simulink model "simpleSwitchWithSubsystemIn"  (R2025a)
settings: Solver=ode4  StartTime=0.0  StopTime=10.0  FixedStep=0.1  RelTol=1e-3
model workspace (MAT data in the model file):
  Bias1 = -2
  Bias2 = -2
  Bias3 = -2
  Bias4 = -2
libraries: simulink x2
settings Model: Creator=The MathWorks, Inc.  LastModifiedBy=The MathWorks, Inc.
settings SolverCC: AlgebraicLoopSolver=TrustRegion
settings DataIOCC: SaveTime=off
settings DebuggingCC: UnconnectedInputMsg=warning  UnconnectedOutputMsg=warning  UnconnectedLineMsg=warning
settings ModelReferenceCC: EnableRefExpFcnMdlSchedulingChecks=on
settings RTWCC: GPUComputeCapability=3.5  DLArmComputeVersion=19.05

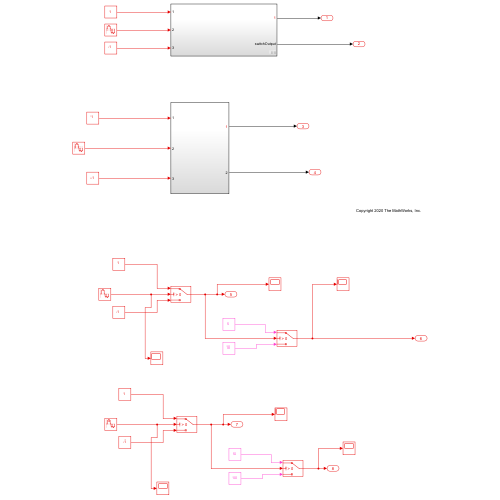
[thumbnail: Simulink's stored preview of the top-level diagram]
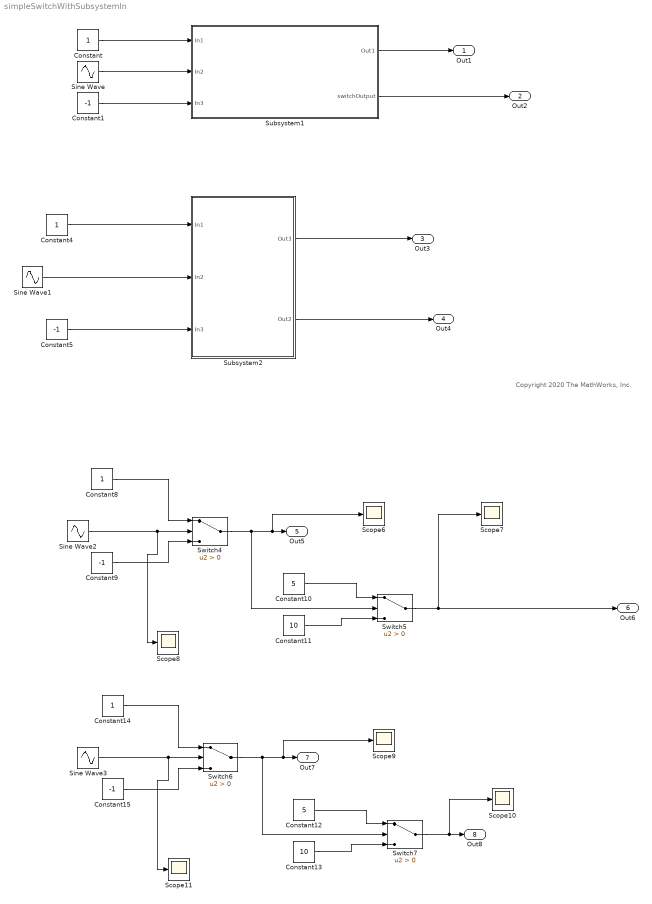
== system simpleSwitchWithSubsystemIn ==
  note: Copyright 2020 The MathWorks, Inc.
  Constant{,4,8,14} (4 alike) : Constant  SampleTime=0.1
  Constant{1,5,9,15} (4 alike) : Constant  Value=-1  SampleTime=0.1
  Constant10 : Constant  Value=5
  Constant11 : Constant  Value=10
  Constant12 : Constant  Value=5
  Constant13 : Constant  Value=10
  Scope{6..11} (6 alike) : Scope
      Scope10 settings: DataLoggingVariableName=ScopeData9
      Scope11 settings: ActiveDisplayYMinimum=-1.24947  ActiveDisplayYMaximum=1.24947  DataLoggingVariableName=ScopeData10
      Scope6 settings: ActiveDisplayYMinimum=-1.1  ActiveDisplayYMaximum=-0.9  DataLoggingVariableName=ScopeData6
      Scope7 settings: DataLoggingVariableName=ScopeData7
      Scope8 settings: ActiveDisplayYMinimum=-1.24947  ActiveDisplayYMaximum=1.24947  DataLoggingVariableName=ScopeData8
      Scope9 settings: ActiveDisplayYMinimum=-1.1  ActiveDisplayYMaximum=-0.9  DataLoggingVariableName=ScopeData11
  Sine Wave : Sin  Bias=Bias1  SampleTime=0.1
  Sine Wave1 : Sin  Bias=Bias2  SampleTime=0.1
  Sine Wave2 : Sin  Bias=Bias3  SampleTime=0.1
  Sine Wave3 : Sin  Bias=Bias4  SampleTime=0.1
  Subsystem1 : Subsystem
  Subsystem2 : Subsystem
  Switch{4..7} (4 alike) : Switch  Criteria=u2 > Threshold  SaturateOnIntegerOverflow=off  InputSameDT=off
  Out1 : Outport  VectorParamsAs1DForOutWhenUnconnected=off
  Out2 : Outport  Port=2  VectorParamsAs1DForOutWhenUnconnected=off
  Out3 : Outport  Port=3  VectorParamsAs1DForOutWhenUnconnected=off
  Out4 : Outport  Port=4  VectorParamsAs1DForOutWhenUnconnected=off
  Out5 : Outport  Port=5  VectorParamsAs1DForOutWhenUnconnected=off
  Out6 : Outport  Port=6  VectorParamsAs1DForOutWhenUnconnected=off
  Out7 : Outport  Port=7  VectorParamsAs1DForOutWhenUnconnected=off
  Out8 : Outport  Port=8  VectorParamsAs1DForOutWhenUnconnected=off
  wires:
  Constant9/1 -> Switch4/3
  Switch4/1 -> Switch5/2, Scope6/1, Out5/1
  Sine Wave2/1 -> Scope8/1, Switch4/2
  Switch5/1 -> Scope7/1, Out6/1
  Constant11/1 -> Switch5/3
  Constant8/1 -> Switch4/1
  Constant10/1 -> Switch5/1
  Constant12/1 -> Switch7/1
  Constant14/1 -> Switch6/1
  Constant13/1 -> Switch7/3
  Switch7/1 -> Scope10/1, Out8/1
  Sine Wave3/1 -> Scope11/1, Switch6/2
  Switch6/1 -> Switch7/2, Scope9/1, Out7/1
  Constant15/1 -> Switch6/3
  Constant/1 -> Subsystem1/1(In1)
  Sine Wave/1 -> Subsystem1/2(In2)
  Constant1/1 -> Subsystem1/3(In3)
  Subsystem1/1(Out1) -> Out1/1
  Subsystem1/2(switchOutput) -> Out2/1
  Constant4/1 -> Subsystem2/1(In1)
  Sine Wave1/1 -> Subsystem2/2(In2)
  Constant5/1 -> Subsystem2/3(In3)
  Subsystem2/1(Out3) -> Out3/1
  Subsystem2/2(Out2) -> Out4/1

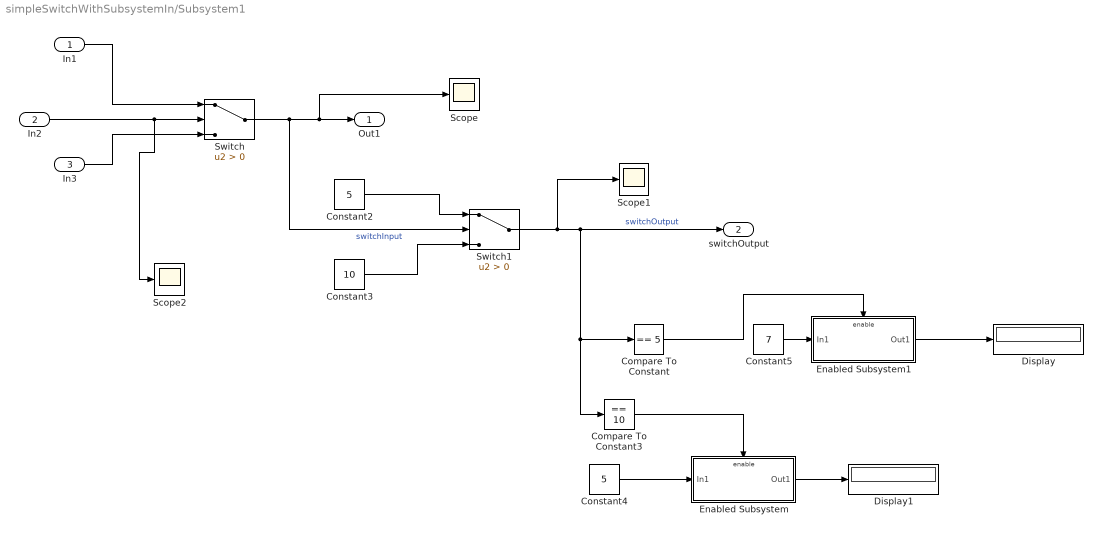
== system simpleSwitchWithSubsystemIn/Subsystem1 ==
  In1 : Inport
  In2 : Inport  Port=2
  In3 : Inport  Port=3
  Compare To Constant : simulink/Logic and Bit Operations/Compare To Constant  relop===  const=5  OutDataTypeStr=boolean
  Compare To Constant3 : simulink/Logic and Bit Operations/Compare To Constant  relop===  const=10  OutDataTypeStr=boolean
  Constant2 : Constant  Value=5
  Constant3 : Constant  Value=10
  Constant4 : Constant  Value=5
  Constant5 : Constant  Value=7
  Display : Display
  Display1 : Display
  Enabled Subsystem : Subsystem  TreatAsAtomicUnit=on
  Enabled Subsystem1 : Subsystem  TreatAsAtomicUnit=on
  Scope : Scope
      settings: ActiveDisplayYMinimum=-1.1  ActiveDisplayYMaximum=-0.9
  Scope1 : Scope
      settings: DataLoggingVariableName=ScopeData2
  Scope2 : Scope
      settings: ActiveDisplayYMinimum=-1.24947  ActiveDisplayYMaximum=1.24947
  Switch : Switch  Criteria=u2 > Threshold  SaturateOnIntegerOverflow=off  InputSameDT=off
  Switch1 : Switch  Criteria=u2 > Threshold  SaturateOnIntegerOverflow=off  InputSameDT=off
  Out1 : Outport  VectorParamsAs1DForOutWhenUnconnected=off
  switchOutput : Outport  Port=2
  wires:
  In1/1 -> Switch/1
  In2/1 -> Scope2/1, Switch/2
  In3/1 -> Switch/3
  Switch/1 -> Switch1/2, Out1/1, Scope/1  "switchInput"
  Constant3/1 -> Switch1/3
  Constant2/1 -> Switch1/1
  Constant5/1 -> Enabled Subsystem1/1(In1)
  Constant4/1 -> Enabled Subsystem/1(In1)
  Switch1/1 -> Compare To Constant/1, Compare To Constant3/1, switchOutput/1, Scope1/1  "switchOutput"
  Compare To Constant3/1 -> Enabled Subsystem/Enable
  Enabled Subsystem1/1(Out1) -> Display/1
  Enabled Subsystem/1(Out1) -> Display1/1
  Compare To Constant/1 -> Enabled Subsystem1/Enable

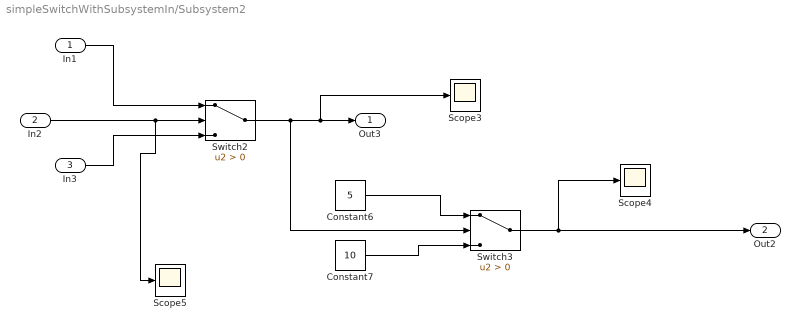
== system simpleSwitchWithSubsystemIn/Subsystem2 ==
  In1 : Inport
  In2 : Inport  Port=2
  In3 : Inport  Port=3
  Constant6 : Constant  Value=5
  Constant7 : Constant  Value=10
  Scope3 : Scope
      settings: ActiveDisplayYMinimum=-1.1  ActiveDisplayYMaximum=-0.9  DataLoggingVariableName=ScopeData3
  Scope4 : Scope
      settings: DataLoggingVariableName=ScopeData4
  Scope5 : Scope
      settings: ActiveDisplayYMinimum=-1.24947  ActiveDisplayYMaximum=1.24947  DataLoggingVariableName=ScopeData5
  Switch2 : Switch  Criteria=u2 > Threshold  SaturateOnIntegerOverflow=off  InputSameDT=off
  Switch3 : Switch  Criteria=u2 > Threshold  SaturateOnIntegerOverflow=off  InputSameDT=off
  Out3 : Outport  VectorParamsAs1DForOutWhenUnconnected=off
  Out2 : Outport  Port=2
  wires:
  In1/1 -> Switch2/1
  Switch3/1 -> Out2/1, Scope4/1
  In2/1 -> Scope5/1, Switch2/2
  Constant6/1 -> Switch3/1
  Constant7/1 -> Switch3/3
  Switch2/1 -> Switch3/2, Out3/1, Scope3/1
  In3/1 -> Switch2/3

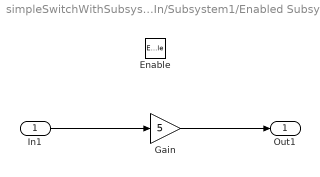
== system simpleSwitchWithSubsystemIn/Subsystem1/Enabled Subsystem ==
  In1 : Inport
  Enable : EnablePort
  Gain : Gain  Gain=5
  Out1 : Outport  VectorParamsAs1DForOutWhenUnconnected=off
  wires:
  In1/1 -> Gain/1
  Gain/1 -> Out1/1

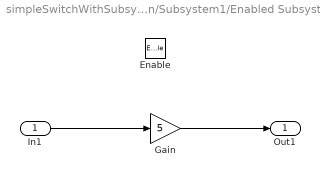
== system simpleSwitchWithSubsystemIn/Subsystem1/Enabled Subsystem1 ==
  In1 : Inport
  Enable : EnablePort
  Gain : Gain  Gain=5
  Out1 : Outport  VectorParamsAs1DForOutWhenUnconnected=off
  wires:
  Gain/1 -> Out1/1
  In1/1 -> Gain/1
